simulink model "HYD21"  (R2018b)
settings: configuration reference "Test_Config" (kept outside this file)
undefined symbols (not defined in the file): EDP_PRESS, ENG_SPD_RPM, FALSE, HI_PRES_THRE, LO_PRES_THRS, TRUE
libraries: simulink x16
(part 2 of 2)

== stateflow chart HYD21/HYD/Locgic_CL ==
  state EDP_DEPRESS [parallel]
    settings: executionOrder=5
    state EDP1ADE [parallel]
      settings: executionOrder=1
      state NORM
        en:
        SYS1_EDP_DE_SW= 0;
      state DE_PRESS
        en:
        SYS1_EDP_DE_SW = 1;
      (default) -> EDP_DEPRESS.EDP1ADE.NORM
      EDP_DEPRESS.EDP1ADE.NORM -> EDP_DEPRESS.EDP1ADE.DE_PRESS : [LENG_STD == 0 &&...
          | LENG_N2 < 15]
      EDP_DEPRESS.EDP1ADE.DE_PRESS -> EDP_DEPRESS.EDP1ADE.NORM : [LENG_N2 > 40 &&...
          | LENG_STD == 2]
    state EDP2ADE [parallel]
      settings: executionOrder=2
      state NORM
        en:
        SYS2_EDP_DE_SW= 0;
      state DE_PRESS
        en:
        SYS2_EDP_DE_SW = 1;
      (default) -> EDP_DEPRESS.EDP2ADE.NORM
      EDP_DEPRESS.EDP2ADE.NORM -> EDP_DEPRESS.EDP2ADE.DE_PRESS : [RENG_STD ==0 &&...
          | RENG_N2 < 15]
      EDP_DEPRESS.EDP2ADE.DE_PRESS -> EDP_DEPRESS.EDP2ADE.NORM : [RENG_N2 > 40 &&...
          | RENG_STD == 2]
  state SYS12_FWSOV [parallel]
    settings: executionOrder=1
    state FWSOV1 [parallel]
      settings: executionOrder=1
      state MAN
        ex:
        EDP_SOV1_OP = 0;
        EDP_SOV1_CL = 0;
        state NORMAL
          en:
          EDP_SOV1_OP = 0;
          EDP_SOV1_CL = 1;
          ex:
          EDP_SOV1_OP = 0;
          EDP_SOV1_CL = 0;
        state SHUTOFF
          en:
          EDP_SOV1_OP = 1;
          EDP_SOV1_CL = 0;
          ex:
          EDP_SOV1_OP = 0;
          EDP_SOV1_CL = 0;
        (default) -> SYS12_FWSOV.FWSOV1.MAN.NORMAL
        SYS12_FWSOV.FWSOV1.MAN.SHUTOFF -> SYS12_FWSOV.FWSOV1.MAN.NORMAL : [EDP1_SHUT_SW == 0]/{after(1,sec)}
        SYS12_FWSOV.FWSOV1.MAN.NORMAL -> SYS12_FWSOV.FWSOV1.MAN.SHUTOFF : [EDP1_SHUT_SW==1 ]/{after(1,sec)}
      state AUTO
        en:
        EDP_SOV1_OP = 1;
        EDP_SOV1_CL = 0;
        ex:
        EDP_SOV1_OP = 0;
        EDP_SOV1_CL = 0;
      (default) -> SYS12_FWSOV.FWSOV1.MAN
      SYS12_FWSOV.FWSOV1.MAN -> SYS12_FWSOV.FWSOV1.AUTO : [SYS1_TEMP>135 ||...
          | LENG_FA]/{after(1,sec)}
      SYS12_FWSOV.FWSOV1.AUTO -> SYS12_FWSOV.FWSOV1.MAN : [SYS1_TEMP < 135 &&...
          | ~LENG_FA]/{after(1,sec)}
    state FWSOV2 [parallel]
      settings: executionOrder=2
      state MAN
        ex:
        EDP_SOV2_OP = 0;
        EDP_SOV2_CL = 0;
        state NORMAL
          en:
          EDP_SOV2_OP = 0;
          EDP_SOV2_CL = 1;
          ex:
          EDP_SOV2_OP = 0;
          EDP_SOV2_CL = 0;
        state SHUTOFF
          en:
          EDP_SOV2_OP = 1;
          EDP_SOV2_CL = 0;
          ex:
          EDP_SOV2_OP = 0;
          EDP_SOV2_CL = 0;
        (default) -> SYS12_FWSOV.FWSOV2.MAN.NORMAL
        SYS12_FWSOV.FWSOV2.MAN.SHUTOFF -> SYS12_FWSOV.FWSOV2.MAN.NORMAL : [EDP2_SHUT_SW == 0]/{after(1,sec)}
        SYS12_FWSOV.FWSOV2.MAN.NORMAL -> SYS12_FWSOV.FWSOV2.MAN.SHUTOFF : [EDP2_SHUT_SW==1 ]/{after(1,sec)}
      state AUTO
        en:
        EDP_SOV2_OP = 1;
        EDP_SOV2_CL = 0;
        ex:
        EDP_SOV2_OP = 0;
        EDP_SOV2_CL = 0;
      (default) -> SYS12_FWSOV.FWSOV2.MAN
      SYS12_FWSOV.FWSOV2.MAN -> SYS12_FWSOV.FWSOV2.AUTO : [SYS2_TEMP>135 ||...
          | RENG_FA]/{after(1,sec)}
      SYS12_FWSOV.FWSOV2.AUTO -> SYS12_FWSOV.FWSOV2.MAN : [SYS2_TEMP < 135 &&...
          | ~RENG_FA]/{after(1,sec)}
  state SYS12_ACMP [parallel]
    settings: executionOrder=2
    state SYS1_ACMP [parallel]
      settings: executionOrder=1
      state VALID
        state OFF
          en:
          ACMP_1B_ST = 0;
        state ON
          en:
          ACMP_1B_ST = 1;
        state AUTO
          state OFF
            en:
            ACMP_1B_ST = 0;
          state ON
            en:
            ACMP_1B_ST = 1;
          (default) -> SYS12_ACMP.SYS1_ACMP.VALID.AUTO.OFF
          SYS12_ACMP.SYS1_ACMP.VALID.AUTO.ON -> SYS12_ACMP.SYS1_ACMP.VALID.AUTO.OFF : [SYS1_TEMP > 135]
          SYS12_ACMP.SYS1_ACMP.VALID.AUTO.OFF -> SYS12_ACMP.SYS1_ACMP.VALID.AUTO.ON : [((TH_HAD_DEG > 53 && WOW == 0) ||...
              |  WOW == 1) && (EDP_1A_PL || ...
              | LENG_N2 <= 60 ||...
              | FLAP_HAD ~= 0)&&...
              | SYS1_TEMP <=135 ||...
              | LENG_STD == 3]
        SYS12_ACMP.SYS1_ACMP.VALID.ON -> SYS12_ACMP.SYS1_ACMP.VALID.OFF [order 1] : [ACMP_1B_SW == 0]
        SYS12_ACMP.SYS1_ACMP.VALID.OFF -> SYS12_ACMP.SYS1_ACMP.VALID.ON [order 2] : [ACMP_1B_SW == 2]
        SYS12_ACMP.SYS1_ACMP.VALID.ON -> SYS12_ACMP.SYS1_ACMP.VALID.AUTO [order 2] : [ACMP_1B_SW == 1]
        SYS12_ACMP.SYS1_ACMP.VALID.AUTO -> SYS12_ACMP.SYS1_ACMP.VALID.ON [order 2] : [ACMP_1B_SW == 2]
        SYS12_ACMP.SYS1_ACMP.VALID.AUTO -> SYS12_ACMP.SYS1_ACMP.VALID.OFF [order 1] : [ACMP_1B_SW == 0]
        SYS12_ACMP.SYS1_ACMP.VALID.OFF -> SYS12_ACMP.SYS1_ACMP.VALID.AUTO [order 1] : [ACMP_1B_SW == 1]
        (default) -> SYS12_ACMP.SYS1_ACMP.VALID.AUTO
      state INVALID
        en:
        ACMP_1B_ST = 2;
      SYS12_ACMP.SYS1_ACMP.INVALID -> SYS12_ACMP.SYS1_ACMP.VALID : [ACMP1B_VALID]
      SYS12_ACMP.SYS1_ACMP.VALID -> SYS12_ACMP.SYS1_ACMP.INVALID : [~ACMP1B_VALID]
      (default) -> SYS12_ACMP.SYS1_ACMP.INVALID
    state SYS2_ACMP [parallel]
      settings: executionOrder=2
      state VALID
        state OFF
          en:
          ACMP_2B_ST = 0;
        state ON
          en:
          ACMP_2B_ST = 1
        state AUTO
          state OFF
            en:
            ACMP_2B_ST = 0;
          state ON
            en:
            ACMP_2B_ST = 1;
          (default) -> SYS12_ACMP.SYS2_ACMP.VALID.AUTO.OFF
          SYS12_ACMP.SYS2_ACMP.VALID.AUTO.ON -> SYS12_ACMP.SYS2_ACMP.VALID.AUTO.OFF : [SYS2_TEMP > 135]
          SYS12_ACMP.SYS2_ACMP.VALID.AUTO.OFF -> SYS12_ACMP.SYS2_ACMP.VALID.AUTO.ON : [((TH_HAD_DEG > 53&& WOW == 0) ||...
              |  WOW == 1) && (EDP_2A_PL || ...
              | RENG_N2 <= 60 ||...
              | FLAP_HAD ~= 0)&&...
              | SYS2_TEMP<=135||...
              | RENG_STD == 3]
        SYS12_ACMP.SYS2_ACMP.VALID.ON -> SYS12_ACMP.SYS2_ACMP.VALID.OFF [order 1] : [ACMP_2B_SW == 0]
        SYS12_ACMP.SYS2_ACMP.VALID.OFF -> SYS12_ACMP.SYS2_ACMP.VALID.ON [order 2] : [ACMP_2B_SW == 2]
        SYS12_ACMP.SYS2_ACMP.VALID.ON -> SYS12_ACMP.SYS2_ACMP.VALID.AUTO [order 2] : [ACMP_2B_SW == 1]
        SYS12_ACMP.SYS2_ACMP.VALID.AUTO -> SYS12_ACMP.SYS2_ACMP.VALID.ON [order 2] : [ACMP_2B_SW == 2]
        SYS12_ACMP.SYS2_ACMP.VALID.AUTO -> SYS12_ACMP.SYS2_ACMP.VALID.OFF [order 1] : [ACMP_2B_SW == 0]
        SYS12_ACMP.SYS2_ACMP.VALID.OFF -> SYS12_ACMP.SYS2_ACMP.VALID.AUTO [order 1] : [ACMP_2B_SW == 1]
        (default) -> SYS12_ACMP.SYS2_ACMP.VALID.AUTO
      state INVALID
        en:
        ACMP_1B_ST = 2;
      SYS12_ACMP.SYS2_ACMP.INVALID -> SYS12_ACMP.SYS2_ACMP.VALID : [ACMP2B_VALID]
      SYS12_ACMP.SYS2_ACMP.VALID -> SYS12_ACMP.SYS2_ACMP.INVALID : [~ACMP2B_VALID]
      (default) -> SYS12_ACMP.SYS2_ACMP.INVALID
  state SYS3_ACMP [parallel]
    settings: executionOrder=3
    state SYS3_ACMP2 [parallel]
      settings: executionOrder=2
      state OFF
        en:
        ACMP_3B_ST = 0;
      state ON
        en:
        ACMP_3B_ST = 1;
      state AUTO
        state OFF
          en:
          ACMP_3A_ST = 0;
          ACMP_3B_ST = 0;
        state MODE1
          state OFF
            en:
            ACMP_3A_ST = 1;
            ACMP_3B_ST = 0;
          state ON
            en:
            ACMP_3A_ST = 0;
            ACMP_3B_ST = 1;
          (default) -> SYS3_ACMP.SYS3_ACMP2.AUTO.MODE1.OFF
          SYS3_ACMP.SYS3_ACMP2.AUTO.MODE1.ON -> SYS3_ACMP.SYS3_ACMP2.AUTO.MODE1.OFF : [mod(DAYS,2)==2]
          SYS3_ACMP.SYS3_ACMP2.AUTO.MODE1.OFF -> SYS3_ACMP.SYS3_ACMP2.AUTO.MODE1.ON : [mod(DAYS,2)==1]
        state MODE2
          state OFF
            en:
            ACMP_3B_ST = 1;
            ACMP_3A_ST = 0;
          state ON
            en:
            ACMP_3A_ST = 1;
            ACMP_3B_ST = 2;
          (default) -> SYS3_ACMP.SYS3_ACMP2.AUTO.MODE2.OFF
          SYS3_ACMP.SYS3_ACMP2.AUTO.MODE2.ON -> SYS3_ACMP.SYS3_ACMP2.AUTO.MODE2.OFF : [ACMP3B_VALID ]
          SYS3_ACMP.SYS3_ACMP2.AUTO.MODE2.OFF -> SYS3_ACMP.SYS3_ACMP2.AUTO.MODE2.ON : [ACMP3B_VALID ]
        (default) -> SYS3_ACMP.SYS3_ACMP2.AUTO.OFF
        SYS3_ACMP.SYS3_ACMP2.AUTO.OFF -> SYS3_ACMP.SYS3_ACMP2.AUTO.MODE1 [order 2] : [WOW == 0 &&...
            | STOP_BRK  &&...
            | RENG_STD == 0 &&...
            | LENG_STD == 0&&...
            | SYS3_TEMP<=135 ]
        SYS3_ACMP.SYS3_ACMP2.AUTO.OFF -> SYS3_ACMP.SYS3_ACMP2.AUTO.MODE2 [order 1] : [(WOW == 1 ||...
            | RENG_N2 > 58 ||...
            | LENG_N2 > 58)&&...
            | SYS3_TEMP<=135]
        SYS3_ACMP.SYS3_ACMP2.AUTO.MODE1 -> SYS3_ACMP.SYS3_ACMP2.AUTO.OFF : [SYS3_TEMP > 135]
        SYS3_ACMP.SYS3_ACMP2.AUTO.MODE2 -> SYS3_ACMP.SYS3_ACMP2.AUTO.OFF : [SYS3_TEMP > 135]
      SYS3_ACMP.SYS3_ACMP2.OFF -> SYS3_ACMP.SYS3_ACMP2.ON [order 1] : [ACMP_3B_SW == 2&&...
          | ACMP_3A_ST == 0]
      SYS3_ACMP.SYS3_ACMP2.ON -> SYS3_ACMP.SYS3_ACMP2.OFF [order 1] : [ACMP_3B_SW == 0]
      SYS3_ACMP.SYS3_ACMP2.ON -> SYS3_ACMP.SYS3_ACMP2.AUTO [order 2] : [ACMP_3B_SW == 1]
      SYS3_ACMP.SYS3_ACMP2.AUTO -> SYS3_ACMP.SYS3_ACMP2.ON [order 2] : [ACMP_3B_SW == 2&&...
          | ACMP_3A_ST == 0]
      SYS3_ACMP.SYS3_ACMP2.AUTO -> SYS3_ACMP.SYS3_ACMP2.OFF [order 1] : [ACMP_3B_SW == 0]
      SYS3_ACMP.SYS3_ACMP2.OFF -> SYS3_ACMP.SYS3_ACMP2.AUTO [order 2] : [ACMP_3B_SW == 1]
      (default) -> SYS3_ACMP.SYS3_ACMP2.AUTO
    state SYS3_ACMP1 [parallel]
      settings: executionOrder=1
      state OFF
        en:
        ACMP_3A_ST = 0;
      state ON
        en:
        ACMP_3A_ST = 1
      state AUTO
        state OFF
          en:
          ACMP_3A_ST = 0;
          ACMP_3B_ST = 0;
        state MODE1
          state OFF
            en:
            ACMP_3A_ST = 1;
            ACMP_3B_ST = 0;
          state ON
            en:
            ACMP_3A_ST = 0;
            ACMP_3B_ST = 1;
          (default) -> SYS3_ACMP.SYS3_ACMP1.AUTO.MODE1.OFF
          SYS3_ACMP.SYS3_ACMP1.AUTO.MODE1.ON -> SYS3_ACMP.SYS3_ACMP1.AUTO.MODE1.OFF : [mod(DAYS,2)==2]
          SYS3_ACMP.SYS3_ACMP1.AUTO.MODE1.OFF -> SYS3_ACMP.SYS3_ACMP1.AUTO.MODE1.ON : [mod(DAYS,2)==1]
        state MODE2
          state OFF
            en:
            ACMP_3A_ST = 1;
            ACMP_3B_ST = 0;
          state ON
            en:
            ACMP_3B_ST = 1;
            ACMP_3A_ST = 2；
          (default) -> SYS3_ACMP.SYS3_ACMP1.AUTO.MODE2.OFF
          SYS3_ACMP.SYS3_ACMP1.AUTO.MODE2.ON -> SYS3_ACMP.SYS3_ACMP1.AUTO.MODE2.OFF : [~ACMP3A_VALID]
          SYS3_ACMP.SYS3_ACMP1.AUTO.MODE2.OFF -> SYS3_ACMP.SYS3_ACMP1.AUTO.MODE2.ON : [ACMP3A_VALID]
        (default) -> SYS3_ACMP.SYS3_ACMP1.AUTO.OFF
        SYS3_ACMP.SYS3_ACMP1.AUTO.OFF -> SYS3_ACMP.SYS3_ACMP1.AUTO.MODE1 [order 2] : [WOW == 0 &&...
            | STOP_BRK  &&...
            | RENG_STD == 0 &&...
            | LENG_STD == 0 &&...
            | SYS3_TEMP<= 135]
        SYS3_ACMP.SYS3_ACMP1.AUTO.MODE1 -> SYS3_ACMP.SYS3_ACMP1.AUTO.OFF : [SYS3_TEMP > 135]
        SYS3_ACMP.SYS3_ACMP1.AUTO.OFF -> SYS3_ACMP.SYS3_ACMP1.AUTO.MODE2 [order 1] : [(WOW == 1 ||...
            | RENG_N2 > 58  ||...
            | LENG_N2 > 58)&&...
            | SYS3_TEMP <= 135]
        SYS3_ACMP.SYS3_ACMP1.AUTO.MODE2 -> SYS3_ACMP.SYS3_ACMP1.AUTO.OFF : [SYS3_TEMP > 135]
      SYS3_ACMP.SYS3_ACMP1.OFF -> SYS3_ACMP.SYS3_ACMP1.ON [order 1] : [ACMP_3A_SW == 2&&...
          | ACMP_3B_ST==0]
      SYS3_ACMP.SYS3_ACMP1.ON -> SYS3_ACMP.SYS3_ACMP1.OFF [order 1] : [ACMP_3A_SW == 0]
      SYS3_ACMP.SYS3_ACMP1.ON -> SYS3_ACMP.SYS3_ACMP1.AUTO [order 2] : [ACMP_3A_SW == 1]
      SYS3_ACMP.SYS3_ACMP1.AUTO -> SYS3_ACMP.SYS3_ACMP1.ON [order 1] : [ACMP_3A_SW == 2&&...
          | ACMP_3B_ST==0]
      SYS3_ACMP.SYS3_ACMP1.OFF -> SYS3_ACMP.SYS3_ACMP1.AUTO [order 2] : [ACMP_3A_SW == 1]
      SYS3_ACMP.SYS3_ACMP1.AUTO -> SYS3_ACMP.SYS3_ACMP1.OFF [order 2] : [ACMP_3A_SW == 0]
      (default) -> SYS3_ACMP.SYS3_ACMP1.AUTO
  state PUV [parallel] [commented out]
    state OFF [commented out]
      en:
      PUV_ST = 0;
  state PTU [parallel]
    settings: executionOrder=4
    state OFF
      en:
      PTU_ST = 0;
    state ON
      en:
      PTU_ST = 1;
    state AUTO
      state OFF
        en:
        PTU_ST = 0;
      state ON
        en:
        PTU_ST = 1;
      (default) -> PTU.AUTO.OFF
      PTU.AUTO -> (junction 485) [order 1]
      (junction 485) -> PTU.AUTO.OFF [order 2]
      (junction 485) -> PTU.AUTO.ON [order 1] : [SYS2_QTY >= 12&&...
          | WOW == 0 &&...
          | (EDP2A_WORK_STD == 1 ||...
          | RENG_STD == 3) &&...
          | EDP1A_WORK_STD == 0&&...
          | (FLAP_HAD ~= 0 ||...
          |  (GEAR_POS~= 0 && GEAR_LOCK == 1))  ]
    note: 起落架不在收上，并锁定位置
    PTU.OFF -> PTU.ON [order 1] : [PTU_SW == 2]
    PTU.ON -> PTU.OFF [order 1] : [PTU_SW == 0]
    PTU.ON -> PTU.AUTO [order 2] : [PTU_SW == 1]
    PTU.AUTO -> PTU.ON [order 1] : [PTU_SW == 2]
    PTU.AUTO -> PTU.OFF [order 2] : [PTU_SW == 0]
    PTU.OFF -> PTU.AUTO [order 2] : [PTU_SW == 1]
    (default) -> PTU.AUTO
  data: EDP1_SHUT_SW input; EDP2_SHUT_SW input; ACMP_1B_SW input; ACMP_2B_SW input; ACMP_3A_SW input; ACMP_3B_SW input; PTU_SW input; TH_HAD_DEG input; FLAP_HAD input; LENG_FA input; RENG_FA input; LENG_STD input; RENG_STD input; LENG_N2 input; RENG_N2 input; STOP_BRK input; WOW input; GEAR_POS input; GEAR_LOCK input; SYS1_TEMP input; SYS2_TEMP input; ACMP_1B_ST output; ACMP_2B_ST output; PTU_ST output; ACMP_3A_ST output; ACMP_3B_ST output; SYS1_EDP_DE_SW output; SYS2_EDP_DE_SW output; EDP_SOV1_OP output; EDP_SOV1_CL output; SYS3_TEMP input; SYS2_QTY input; EDP_2A_PL input; EDP_1A_PL input; DAYS input; ACMP1B_VALID input; ACMP2B_VALID input; EDP_SOV2_OP output; EDP_SOV2_CL output; ACMP3A_VALID input; ACMP3B_VALID input; EDP1A_WORK_STD input; EDP2A_WORK_STD input
